simulink model "hw3_p2_Boeing727"  (R2020a)
settings: Solver=VariableStepAuto  StartTime=0.0  StopTime=1500  RelTol=1e-12
undefined symbols (not defined in the file or in its folder): alpha_i, beta_i, da, dr, dT, dtheta, h0, u0
settings Model: Creator=Tomo  LastModifiedBy=Tomo

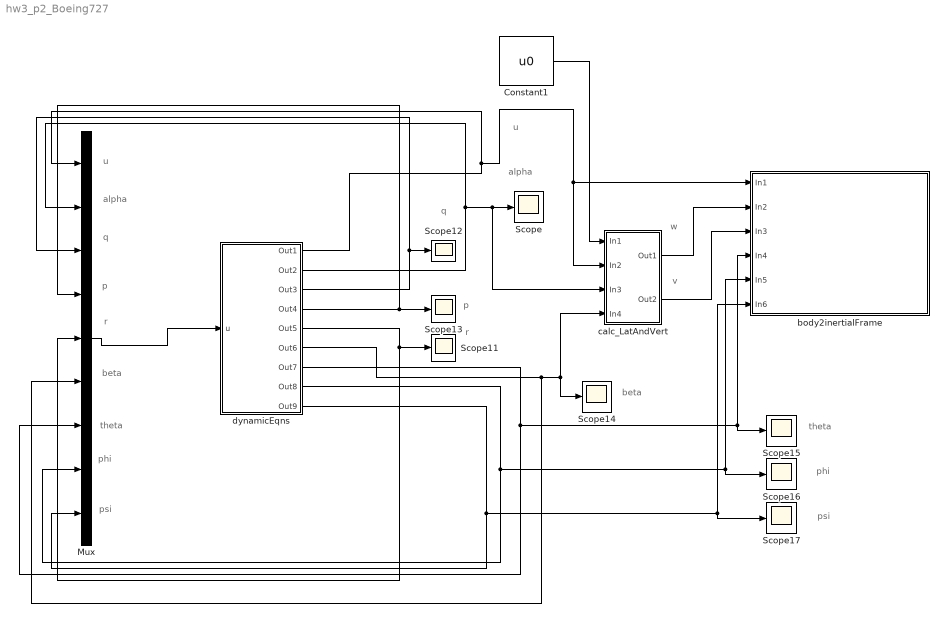
== system hw3_p2_Boeing727 ==
  note: alpha
  note: q
  note: p
  note: r
  note: beta
  note: theta
  note: phi
  note: psi
  note: v
  note: w
  note: u
  note: u
  note: alpha
  note: q
  note: p
  note: r
  note: beta
  note: theta
  note: phi
  note: psi
  Constant1 : Constant  Value=u0
  Mux : Mux  Inputs=9
  Scope{,11..17} (8 alike) : Scope
  body2inertialFrame : Subsystem
  calc_LatAndVert : Subsystem
  dynamicEqns : Subsystem
  wires:
  dynamicEqns/9(Out9) -> Mux/9, Scope17/1, body2inertialFrame/6(In6)
  dynamicEqns/8(Out8) -> Mux/8, Scope16/1, body2inertialFrame/5(In5)
  dynamicEqns/7(Out7) -> Mux/7, Scope15/1, body2inertialFrame/4(In4)
  dynamicEqns/6(Out6) -> Mux/6, Scope14/1, calc_LatAndVert/4(In4)
  dynamicEqns/5(Out5) -> Mux/5, Scope11/1
  dynamicEqns/4(Out4) -> Mux/4, Scope13/1
  dynamicEqns/3(Out3) -> Mux/3, Scope12/1
  dynamicEqns/2(Out2) -> Mux/2, Scope/1, calc_LatAndVert/3(In3)
  dynamicEqns/1(Out1) -> Mux/1, body2inertialFrame/1(In1), calc_LatAndVert/2(In2)
  Mux/1 -> dynamicEqns/1(u)
  Constant1/1 -> calc_LatAndVert/1(In1)
  calc_LatAndVert/1(Out1) -> body2inertialFrame/2(In2)
  calc_LatAndVert/2(Out2) -> body2inertialFrame/3(In3)

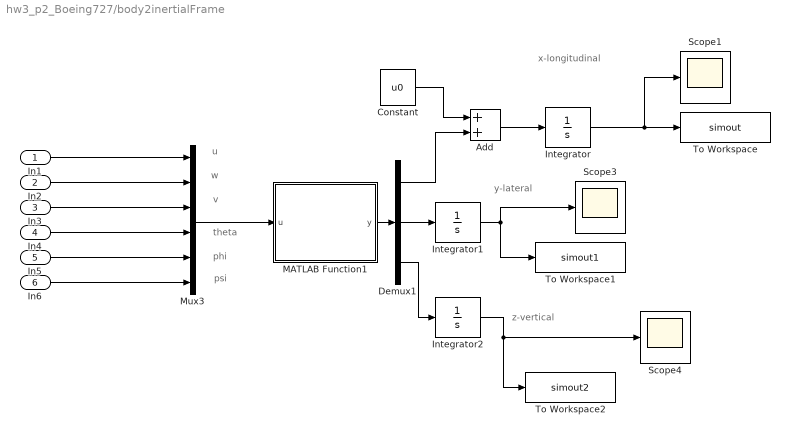
== system hw3_p2_Boeing727/body2inertialFrame ==
  note: x-longitudinal
  note: y-lateral
  note: z-vertical
  note: u
  note: w
  note: v
  note: theta
  note: phi
  note: psi
  In1 : Inport
  In2 : Inport  Port=2
  In3 : Inport  Port=3
  In4 : Inport  Port=4
  In5 : Inport  Port=5
  In6 : Inport  Port=6
  Add : Sum
  Constant : Constant  Value=u0
  Demux1 : Demux  Outputs=3
  Integrator : Integrator
  Integrator1 : Integrator
  Integrator2 : Integrator  InitialCondition=h0
  MATLAB Function1 : MATLAB Function  TreatAsAtomicUnit=on
  Mux3 : Mux  Inputs=6
  Scope1 : Scope
  Scope3 : Scope
  Scope4 : Scope
  To Workspace : ToWorkspace  VariableName=simout  SaveFormat=Structure With Time  SampleTime=-1
  To Workspace1 : ToWorkspace  VariableName=simout1  SaveFormat=Structure With Time  SampleTime=-1
  To Workspace2 : ToWorkspace  VariableName=simout2  SaveFormat=Structure With Time  SampleTime=-1
  wires:
  Integrator2/1 -> To Workspace2/1, Scope4/1
  Integrator/1 -> Scope1/1, To Workspace/1
  In2/1 -> Mux3/2
  Mux3/1 -> MATLAB Function1/1(u)
  Integrator1/1 -> Scope3/1, To Workspace1/1
  In4/1 -> Mux3/4
  MATLAB Function1/1(y) -> Demux1/1
  Demux1/3 -> Integrator2/1
  Demux1/2 -> Integrator1/1
  In1/1 -> Mux3/1
  In5/1 -> Mux3/5
  In6/1 -> Mux3/6
  In3/1 -> Mux3/3
  Constant/1 -> Add/1
  Demux1/1 -> Add/2
  Add/1 -> Integrator/1

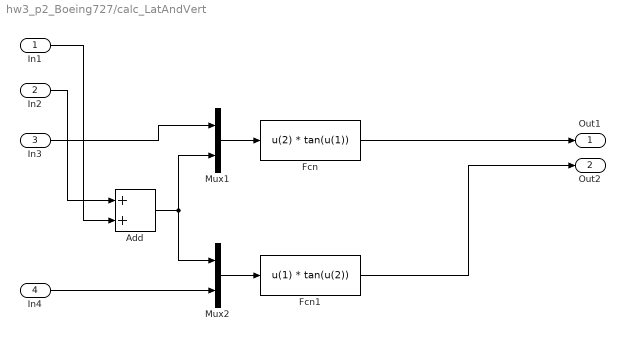
== system hw3_p2_Boeing727/calc_LatAndVert ==
  In1 : Inport
  In2 : Inport  Port=2
  In3 : Inport  Port=3
  In4 : Inport  Port=4
  Add : Sum
  Fcn : Fcn  Expr=u(2) * tan(u(1))
  Fcn1 : Fcn  Expr=u(1) * tan(u(2))
  Mux1 : Mux  Inputs=2
  Mux2 : Mux  Inputs=2
  Out1 : Outport
  Out2 : Outport  Port=2
  wires:
  Mux1/1 -> Fcn/1
  Add/1 -> Mux2/1, Mux1/2
  Mux2/1 -> Fcn1/1
  In1/1 -> Add/2
  In3/1 -> Mux1/1
  Fcn/1 -> Out1/1
  In4/1 -> Mux2/2
  Fcn1/1 -> Out2/1
  In2/1 -> Add/1

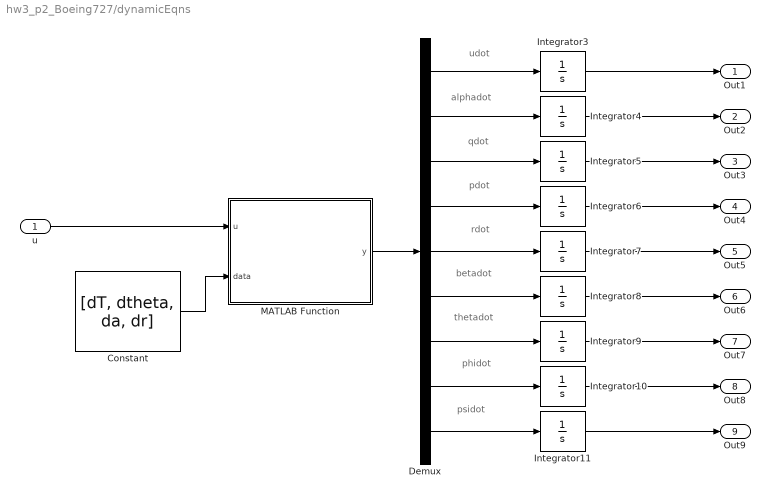
== system hw3_p2_Boeing727/dynamicEqns ==
  note: udot
  note: alphadot
  note: qdot
  note: pdot
  note: rdot
  note: betadot
  note: thetadot
  note: phidot
  note: psidot
  u : Inport
  Constant : Constant  Value=[dT, dtheta, da, dr]
  Demux : Demux  Outputs=9
  Integrator{3,5..7,9..11} (7 alike) : Integrator
  Integrator4 : Integrator  InitialCondition=alpha_i
  Integrator8 : Integrator  InitialCondition=beta_i
  MATLAB Function : MATLAB Function  TreatAsAtomicUnit=on
  Out1 : Outport
  Out2 : Outport  Port=2
  Out3 : Outport  Port=3
  Out4 : Outport  Port=4
  Out5 : Outport  Port=5
  Out6 : Outport  Port=6
  Out7 : Outport  Port=7
  Out8 : Outport  Port=8
  Out9 : Outport  Port=9
  wires:
  Integrator5/1 -> Out3/1
  Integrator9/1 -> Out7/1
  Demux/2 -> Integrator4/1
  Demux/6 -> Integrator8/1
  Demux/1 -> Integrator3/1
  Constant/1 -> MATLAB Function/2(data)
  Integrator3/1 -> Out1/1
  Demux/8 -> Integrator10/1
  Demux/4 -> Integrator6/1
  Demux/3 -> Integrator5/1
  Demux/7 -> Integrator9/1
  Demux/5 -> Integrator7/1
  Demux/9 -> Integrator11/1
  u/1 -> MATLAB Function/1(u)
  MATLAB Function/1(y) -> Demux/1
  Integrator4/1 -> Out2/1
  Integrator10/1 -> Out8/1
  Integrator7/1 -> Out5/1
  Integrator6/1 -> Out4/1
  Integrator8/1 -> Out6/1
  Integrator11/1 -> Out9/1

== matlab function hw3_p2_Boeing727/dynamicEqns/MATLAB Function ==
  data: u input size=9; y output size=9; data input size=4
function y = fcn(u, data)
    % Unpack the delta inputs 
    dT = data(1); dtheta = data(2); da = data(3); dr = data(4);
    % Unpack the input variables 
    uv = u(1); alpha = u(2); q = u(3); p = u(4); r = u(5);
    beta = u(6); theta = u(7); phi = u(8); psi = u(9);
    
    % Functions 
    alphadot = -0.0001*uv -0.9967*alpha +1.0046*q +0.03867*(cos(theta)*cos(phi)-1.0)...
                -0.03827*dtheta;
    betadot  = -0.2127*beta -0.0011*p -0.9957*r +0.03867*cos(theta)*sin(phi)...
                +0.03259*dr;
    udot     = -0.01008*uv +2.425*alphadot +7.055*alpha -2.308*q -32.17*theta...
                -0.9679*dtheta +0.004*dT;
    qdot     = 0.8277*alphadot -0.000013*uv -3.326*alpha -1.337*q -2.57*dtheta;
    pdot     = -2.5612*p +0.7245*r -0.0677*betadot -14.0174*beta +0.4395*da +0.3830*dr;
    rdot     = 0.8476*p -0.4155*r +0.3564*betadot +6.6931*beta -0.1556*da -0.7090*dr;
    thetadot = q*cos(phi) - r*sin(phi);
    phidot   = p + q*sin(phi)*tan(theta) + r*cos(phi)*tan(theta);
    psidot   = (q*sin(phi) + r*cos(phi))*sec(theta);
    
    y = [udot; alphadot; qdot; pdot; rdot; betadot; thetadot; phidot; psidot];
end

== matlab function hw3_p2_Boeing727/body2inertialFrame/MATLAB Function1 ==
  data: u input size=6; y output size=3
function y = fcn(u)
    % Rotation transformation from body-frame to inertial-frame
    uv = u(1); wv = u(2); vv = u(3);
    theta = u(4); phi = u(5); psi = u(6);
    
    R3 = [cos(psi), -sin(psi), 0;
          sin(psi),  cos(psi), 0;
                 0,         0, 1];
    R2 = [ cos(theta), 0, sin(theta);
                    0, 1,          0;
          -sin(theta), 0, cos(theta)];
    R1 = [1,        0,         0;
          0, cos(phi), -sin(phi);
          0, sin(phi),  cos(phi)];
    y = R3*R2*R1 * [uv; vv; wv];  
end
